simulink library "Lib_DQTrans_abc2dqs"  (R2021a)
settings: Solver=VariableStepAuto  StartTime=0.0  StopTime=10.0  RelTol=1e-3
undefined symbols (not defined in the file): C_INV_N3, C_INV_SQRT3
settings Model: Creator=30610  LastModifiedBy=30610

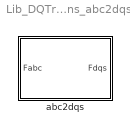
== system Lib_DQTrans_abc2dqs ==
  abc2dqs : Subsystem  Description=DQ Transformation

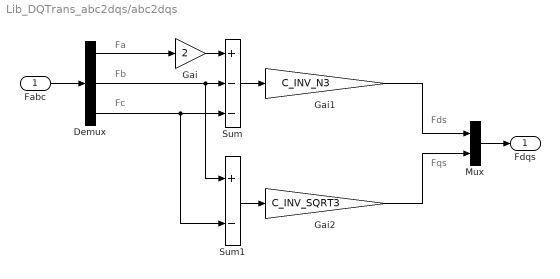
== system Lib_DQTrans_abc2dqs/abc2dqs ==
  note: Fqs
  note: Fds
  note: Fa
  note: Fb
  note: Fc
  Fabc : Inport  OutDataTypeStr=single
  Demux : Demux  Outputs=3
  Gai : Gain  Gain=2
  Gai1 : Gain  Gain=C_INV_N3
  Gai2 : Gain  Gain=C_INV_SQRT3
  Mux : Mux  Inputs=2
  Sum : Sum  Inputs=+--
  Sum1 : Sum  Inputs=+-
  Fdqs : Outport  OutDataTypeStr=single  VectorParamsAs1DForOutWhenUnconnected=off
  wires:
  Demux/2 -> Sum1/1, Sum/2
  Mux/1 -> Fdqs/1
  Fabc/1 -> Demux/1
  Gai2/1 -> Mux/2
  Gai1/1 -> Mux/1
  Sum1/1 -> Gai2/1
  Sum/1 -> Gai1/1
  Demux/3 -> Sum1/2, Sum/3
  Gai/1 -> Sum/1
  Demux/1 -> Gai/1
